simulink model "Task3_GradingSystem"  (R2021a)
settings: Solver=FixedStepDiscrete  StartTime=0.0  StopTime=10.0  RelTol=1e-3  EnableMultiTasking=on
settings Model: SILPILModeSetting=veronly  ExtModeTrigDuration=2  Creator=Michael_Ibrahim  LastModifiedBy=Michael_Ibrahim
settings DataIOCC: ReturnWorkspaceOutputs=off
settings OptimizationCC: EnableMemcpy=off  LifeSpan=1  MaxStackSize=64  EfficientTunableParamExpr=on
settings DebuggingCC: UnderspecifiedInitializationDetection=Classic  MergeDetectMultiDrivingBlocksExec=none  SFMachineParentedDataDiag=warning  ArithmeticOperatorsInVariantConditions=warning
settings HardwareCC: ProdBitPerInt=16  ProdBitPerPointer=16  ProdBitPerSizeT=16  ProdBitPerPtrDiffT=16  ProdLargestAtomicFloat=None  ProdWordSize=8  ProdHWDeviceType=Atmel->AVR
settings ModelReferenceCC: PropagateSignalLabelsOutOfModel=off
settings SFSimCC: MATLABDynamicMemAlloc=off  CustomCodeUndefinedFunction=UseInterfaceOnly
settings RTWCC: SystemTargetFile=ert.tlc  HardwareBoard=Arduino Uno  GenCodeOnly=on  TemplateMakefile=ert_default_tmf  GenerateReport=on  Toolchain=Arduino AVR  IncludeHyperlinkInReport=on  LaunchReport=on  GenerateTraceInfo=on  GenerateTraceReport=on  GenerateTraceReportSl=on  GenerateTraceReportSf=on  GenerateTraceReportEml=on
settings CodeAppCC: ForceParamTrailComments=on  IgnoreCustomStorageClasses=off  OperatorAnnotations=on  SimulinkDataObjDesc=on  SFDataObjDesc=on  MATLABFcnDesc=on  InsertBlockDesc=on  StateflowObjectComments=on  MATLABSourceComments=on
settings ERTTargetCC: MultiwordLength=2048  SupportContinuousTime=on  SupportVariableSizeSignals=on  ExtModeStaticAllocSize=250

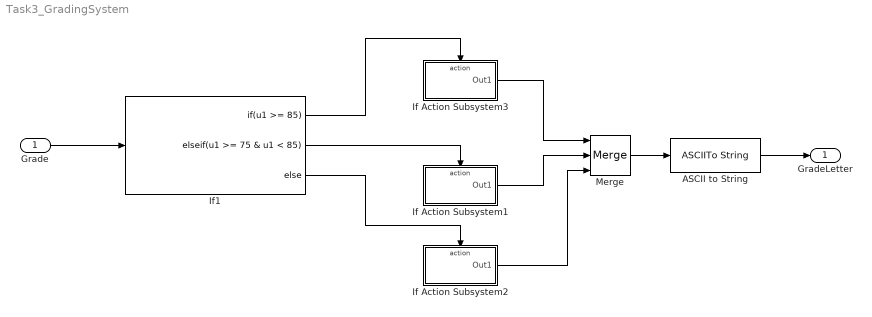
== system Task3_GradingSystem ==
  Grade : Inport
  ASCII to String : ASCIIToString
  If Action Subsystem1 : Subsystem  TreatAsAtomicUnit=on
  If Action Subsystem2 : Subsystem  TreatAsAtomicUnit=on
  If Action Subsystem3 : Subsystem  TreatAsAtomicUnit=on
  If1 : If  IfExpression=u1 >= 85  ElseIfExpressions=u1 >= 75 & u1 < 85
  Merge : Merge  Inputs=3
  GradeLetter : Outport
  wires:
  If1/1 -> If Action Subsystem3/Action
  If1/2 -> If Action Subsystem1/Action
  If1/3 -> If Action Subsystem2/Action
  Grade/1 -> If1/1
  If Action Subsystem3/1(Out1) -> Merge/1
  If Action Subsystem1/1(Out1) -> Merge/2
  If Action Subsystem2/1(Out1) -> Merge/3
  Merge/1 -> ASCII to String/1
  ASCII to String/1 -> GradeLetter/1

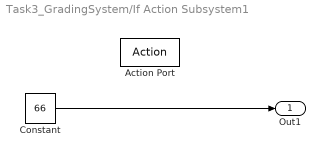
== system Task3_GradingSystem/If Action Subsystem1 ==
  Action Port : ActionPort  ActionPortLabel=elseif(u1 >= 75 & u1 < 85)
  Constant : Constant  Value=66  OutDataTypeStr=uint8
  Out1 : Outport  OutDataTypeStr=uint8
  wires:
  Constant/1 -> Out1/1

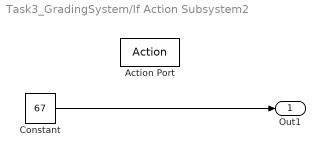
== system Task3_GradingSystem/If Action Subsystem2 ==
  Action Port : ActionPort  ActionPortLabel=else
  Constant : Constant  Value=67  OutDataTypeStr=uint8
  Out1 : Outport  OutDataTypeStr=uint8
  wires:
  Constant/1 -> Out1/1

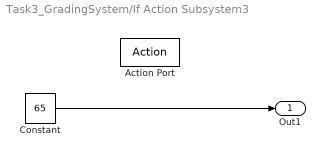
== system Task3_GradingSystem/If Action Subsystem3 ==
  Action Port : ActionPort  ActionPortLabel=if(u1 >= 85)
  Constant : Constant  Value=65  OutDataTypeStr=uint8
  Out1 : Outport  OutDataTypeStr=uint8
  wires:
  Constant/1 -> Out1/1
